simulink model "main_state_v3"  (R2021b)
settings: Solver=VariableStepAuto  StartTime=0.0  StopTime=inf  RelTol=1e-3
undefined symbols (not defined in the file): X, Y, Z
libraries: sm_lib x35, nesl_utility x19, simulink x11, fl_lib x6, ee_lib x3, slpidlib x1
(part 3 of 3)

== stateflow chart main_state_v3/BMS scheduler ==
  state Error_ack_Computer
    error_monitor = 1;
    exit:
    t = 0;
  state emergency
    state Power_management
      if Sys_Amp <= 50 && Over_Amp_Stat==1
      Over_Amp_Stat = 0;
      Emer_Trig = 0;
      elseif Sys_Volt < 24 && Over_Volt_Stat == 1
      Over_Volt_Stat = 0;
      Emer_Trig = 0;
      elseif Sys_Volt > 5 && Under_Volt_Stat ==1
      Under_Volt_Stat = 0;
      Emer_Trig = 0;
      end
    (default) -> emergency.Power_management
  state Power_off
    Time_ack_threshold = 10;
  state Start
    t = 0;
    error_monitor = 0;
    send_heartbeat = 0;
  state ready_Power_on
    du:
    t = t +0.2;
    exit:
    t = 0;
    error_monitor = 0;
  state working
    en:
    Emer_Trig = 0;
    Over_Volt_Stat = 0;
    Under_Volt_Stat = 0;
    Over_Amp_Stat = 0;
    state Power_management
      if Sys_Amp >= 50
      Over_Amp_Stat = 1;
      Emer_Trig = 1;
      elseif Sys_Volt >= 24
      Over_Volt_Stat = 1;
      Emer_Trig = 2;
      elseif Sys_Volt <= 5
      Under_Volt_Stat = 1;
      Emer_Trig = 2;
      end
      state init
        en:
        start_send = 1;
        task = 0;
        send_heartbeat = 1;
      state Charging
        en:
        %start_send = 1;
        task = 1;
      state discharged
        en:
        %start_send = 1;
        task = 1;
      (default) -> init
      Charging -> init : [Batt_percent == 100]
      init -> Charging [order 1] : [Batt_percent  <= 20]
      discharged -> init
      init -> discharged [order 2]
    (default) -> working.Power_management
  state delay_on_device
    en:
    Power_Enable = 1;
    du:
    t = t +0.2;
    exit:
    t = 0;
  note: Computer :on
      | Mcu :on
      | BmsMcu :on
      | By Circuit
  state check_Power_sw
    du:
    t =t +0.2;
    exit:
    t = 0;
  state Send_command_to_Com
    du:
    t = t +0.2;
    exit:
    t = 0;
  note: ส่ง digital_logic ไปยังวงจรจ่ายไฟ
      | ของ Bms_Mcu
  state BMS_Mcu_Power_off
    exit:
    t = 0;
  state turn_off_state
    start_send = 1;
    du:
    t = t +0.2;
    en:
    Com_turn_off = 1;
    exit:
    t = 0;
    start_send = 0;
  state Cut_off_Power_Mcu_Com
    Power_Enable = 0;
    du:
    t = t +0.2;
  state Power_off_check
    ;
  note: Computer Power <= 100mA
  note: Send signal to turn off
      | Mcu, Motor , Computer
  Error_ack_Computer -> Power_off
  ready_Power_on -> Error_ack_Computer [order 2] : [t >= Time_ack_threshold]
  working -> emergency [order 1] : [Emer_Sw_Stat ==1 || Emer_Trig >= 1]
  emergency -> working : [Emer_Sw_Stat == 0&& Emer_Trig== 0]
  (default) -> Start
  ready_Power_on -> delay_on_device [order 1] : [ack_computer == 1]
  delay_on_device -> working : [t>=5]
  Start -> Power_off
  Power_off -> ready_Power_on : [Power_On_Sw_Stat == 1]
  (junction 66) -> working [order 1] : [t <= 3]
  Send_command_to_Com -> working [order 1] : [t >= Time_ack_threshold]
  BMS_Mcu_Power_off -> Power_off
  working -> check_Power_sw [order 2] : [Power_On_Sw_Stat == 1]
  check_Power_sw -> (junction 66) : [Power_On_Sw_Stat==0]
  (junction 66) -> Send_command_to_Com [order 2] : [t>=3]
  Send_command_to_Com -> turn_off_state [order 2] : [ack_computer == 2]
  Cut_off_Power_Mcu_Com -> BMS_Mcu_Power_off : [t>=2]
  turn_off_state -> Power_off_check : [t>=20]
  Power_off_check -> Cut_off_Power_Mcu_Com
  data: ack_computer input; Power_On_Sw_Stat input; Emer_Sw_Stat input; Batt_percent input; start_send output; Batt_data input; task output; Power_Enable output; Time_ack_threshold local; t local; error_monitor output; Com_turn_off output; Sys_Volt input; Sys_Amp input; Over_Volt_Stat local; Under_Volt_Stat local; Over_Amp_Stat local; Emer_Trig output; send_heartbeat output

== stateflow chart main_state_v3/amr scheduler ==
  state Start
    send_heartbeat = 0;
    status = 0;
  state init
  state calibrate
  state emergency
    en:
    status = -1;
    state resume_behavior
      if (Min_Env_Temp_Threshold <Current_Env_Temp)&&(Max_Env_Temp_Threshold  > Current_Env_Temp)
      emer_trig = 0;
      end
  state working
    Max_Env_Temp_Threshold = 40;
    Min_Env_Temp_Threshold = 20;
    state Resume
      if Current_Env_Temp >= Max_Env_Temp_Threshold
      Over_Temp_Stat = 1;
      elseif Current_Env_Temp <= Min_Env_Temp_Threshold
      Under_Temp_Stat = 1;
      end
      en:
      monitor = 0;
      Under_Temp_Stat = 0;
      Over_Temp_Stat = 0;
      emer_trig = 0;
      state init
        en:
        status = 1;
        send_heartbeat = 1;
      state follow_geometry
        en:
        status = 2;
      (default) -> working.Resume.init
      follow_geometry -> working.Resume.init
      working.Resume.init -> follow_geometry : [software_input == 1]
    state Emergency_Trigger
      en:
      emer_trig = 1;
      %send_heartbeat = 0;
      state emer_monitor
        en:
        if Over_Temp_Stat ==1 || Under_Temp_Stat == 1
        monitor = 2 ;
        elseif emer_sig == 1
        monitor = 1 ;
        end
    (default) -> Resume
    Emergency_Trigger -> Resume : [Under_Temp_Stat == 0 &&Over_Temp_Stat == 0]
    Resume -> Emergency_Trigger : [Under_Temp_Stat == 1 ||Over_Temp_Stat == 1 || emer_sig == 1]
  (default) -> Start
  (junction 59) -> Start : [Power_Enable == 0]
  Start -> init : [Power_Enable == 1]
  emergency -> init [order 1] : [emer_sig == 0&&emer_trig == 0]
  init -> calibrate
  calibrate -> working
  working -> (junction 59) [order 2]
  emergency -> (junction 59) [order 2]
  working -> emergency [order 1] : [emer_trig == 1]
  data: Power_Enable input; Current_Env_Temp input; emer_sig input; emer_trig local; Over_Temp_Stat local; Under_Temp_Stat local; Max_Env_Temp_Threshold local; Min_Env_Temp_Threshold local; monitor output; software_input input; status output; send_heartbeat output

== stateflow chart main_state_v3/loop send info2 ==
  state send
    en:
    Batt_monitoring = Batt_data;
    Command_turnoff = Com_turn_off;
    exit:
    Batt_monitoring = 0;
    Command_turnoff = 0;
  state init
  (default) -> init
  init -> send : [start_send ==1]
  send -> init : after(100,msec)
  data: start_send input; Com_turn_off input; Batt_monitoring output; Batt_data input; Command_turnoff output

== stateflow chart main_state_v3/interup send heartbeat3 ==
  state send
    en:
    heartbeat_sig = 1;
  state init
    en:
    heartbeat_sig = 0
  (default) -> init
  init -> send : [send_heartbeat ==1]
  send -> init : after(100,msec)
  data: send_heartbeat input; heartbeat_sig output

== stateflow chart main_state_v3/Heartbeat_protocol2 ==
  state wait_msg
    en:
    t = timer;
  state emer_trig
    en:
    emer_sig = 1;
  state reply_msg
    en:
    reply_msg = 1;
  (default) -> wait_msg : {Heartbeat_Time_Threshold = 2}
  wait_msg -> (junction 49)
  reply_msg -> wait_msg : [after(300,msec)]
  (junction 49) -> emer_trig [order 1] : [ timer - t >= Heartbeat_Time_Threshold]
  (junction 49) -> reply_msg [order 2] : [send_msg == 1]
  data: timer input; reply_msg output; send_msg input; msg local; t local; Heartbeat_Time_Threshold local; emer_sig output

== stateflow chart main_state_v3/Heartbeat_protocol3 ==
  state Start_heartbeat
    en:
    send_msg = 1;
    t = timer;
  state wait_ack
    en:
    t = timer;
  state send_msg
    en:
    send_msg = 1;
  state emer_trig
    en:
    emer_sig = 1;
  (default) -> Start_heartbeat : {Heartbeat_Time_Threshold = 2}
  Start_heartbeat -> wait_ack
  wait_ack -> (junction 48)
  send_msg -> wait_ack : [after(100,msec)]
  (junction 48) -> emer_trig [order 1] : [timer - t >= Heartbeat_Time_Threshold]
  (junction 48) -> send_msg [order 2] : [reply_msg == 1]
  data: timer input; reply_msg input; send_msg output; t local; Heartbeat_Time_Threshold local; emer_sig output

== stateflow chart main_state_v3/EX. Electronic Devices2/Heartbeat_protocol1 ==
  state wait_msg
    en:
    t = timer;
  state emer_trig
    en:
    emer_sig = 1;
    reply_msg = 0;
    exit:
    emer_sig = 0;
  state reply_msg
    en:
    reply_msg = 1;
  (default) -> wait_msg : {Heartbeat_Time_Threshold = 2}
  emer_trig -> wait_msg : [send_msg == 1]
  wait_msg -> (junction 49)
  reply_msg -> wait_msg : [after(300,msec)]
  (junction 49) -> reply_msg [order 2] : [send_msg == 1]
  (junction 49) -> emer_trig [order 1] : [ timer - t >= Heartbeat_Time_Threshold && send_msg==0]
  data: timer input; reply_msg output; send_msg input; msg local; t local; Heartbeat_Time_Threshold local; emer_sig output

== stateflow chart main_state_v3/Heartbeat_protocol4 ==
  state Start
    send_msg = 0;
  state heartbeat
    en:
    send_msg = 1;
    t = timer;
  state wait_ack
    en:
    t = timer;
  state send_msg
    en:
    send_msg = 1;
  state emer_trig
    en:
    emer_sig = 1;
    exit:
    emer_sig = 0;
  (default) -> Start : {Heartbeat_Time_Threshold = 2;}
  (junction 63) -> Start : [heartbeat == 0]
  Start -> heartbeat : [heartbeat == 1]
  heartbeat -> wait_ack
  wait_ack -> (junction 63) [order 1]
  emer_trig -> (junction 63) [order 2]
  emer_trig -> wait_ack [order 1] : [reply_msg == 1]
  wait_ack -> (junction 48) [order 2]
  send_msg -> wait_ack : [after(100,msec)]
  (junction 48) -> emer_trig [order 1] : [timer - t >= Heartbeat_Time_Threshold]
  (junction 48) -> send_msg [order 2] : [reply_msg == 1]
  data: heartbeat input; timer input; reply_msg input; send_msg output; t local; Heartbeat_Time_Threshold local; emer_sig output
